simulink model "milestone3simulink"  (R2020a)
settings: Solver=VariableStepAuto  StartTime=0.0  StopTime=500  RelTol=1e-3
values from neighbouring files (symbols this model uses):
  ac = A-bc*C    [milestone3constants.m]
  alpha_initial = -theta+atan2(dy,dx)    [milestone3constants.m]
  bc = bc_1'    [milestone3constants.m]
  Beq = 0.2963    [milestone3constants.m]
  beta_initial = -theta-alpha_initial    [milestone3constants.m]
  del_weight = 1    [milestone3constants.m]
  g = 9.81    [milestone3constants.m]
  Jeq = 0.01802    [milestone3constants.m]
  k = place(A,B,p)    [milestone3constants.m]
  k_z = B-bc*D    [milestone3constants.m]
  Kb = 2.2179e-3    (= 0.0022179)    [milestone3constants.m]
  Keq = 0.74    [milestone3constants.m]
  mu = 0.01    [milestone3constants.m]
  p_initial = sqrt(dx^2+dy^2)    [milestone3constants.m]
  pick_up = 100    [milestone3constants.m]
  r = 0.037    [milestone3constants.m]
  ra = 7.4    [milestone3constants.m]
  un = [0 0]    [milestone3constants.m]
  v_i = 0    [milestone3constants.m]
  v_o = 0    [milestone3constants.m]
  wl_initial = 0    [milestone3constants.m]
  Wr = 0.18    [milestone3constants.m]
  wr_initial = 0    [milestone3constants.m]
  x_initial = [p_initial alpha_initial beta_initial 3.3275 3.3275]    [milestone3constants.m]
  yn = zeros(1,3)    [milestone3constants.m]
settings Model: Creator=oliviaball  LastModifiedBy=oliviaball
settings DataIOCC: MaxDataPoints=400  ReturnWorkspaceOutputs=off
settings DebuggingCC: ArithmeticOperatorsInVariantConditions=warning
settings SFSimCC: CustomCodeUndefinedFunction=UseInterfaceOnly

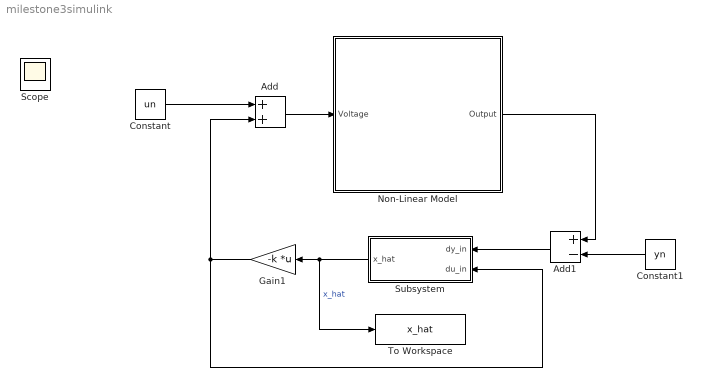
== system milestone3simulink ==
  Add : Sum
  Add1 : Sum  Inputs=+-
  Constant : Constant  Value=un
  Constant1 : Constant  Value=yn
  Gain1 : Gain  Gain=-k  Multiplication=Matrix(K*u)
  Non-Linear Model : Subsystem
  Subsystem : Subsystem
  To Workspace : ToWorkspace  VariableName=x_hat  SaveFormat=Timeseries  SampleTime=-1
  Scope : Scope
  wires:
  Add/1 -> Non-Linear Model/1(Voltage)
  Gain1/1 -> Subsystem/2(du_in), Add/2
  Constant/1 -> Add/1
  Non-Linear Model/1(Output) -> Add1/1
  Constant1/1 -> Add1/2
  Subsystem/1(x_hat) -> To Workspace/1, Gain1/1  "x_hat"
  Add1/1 -> Subsystem/1(dy_in)

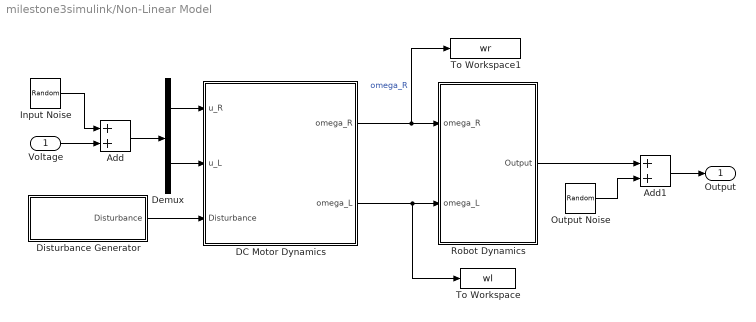
== system milestone3simulink/Non-Linear Model ==
  Voltage : Inport
  Add : Sum
  Add1 : Sum
  DC Motor Dynamics : Subsystem
  Demux : Demux  Outputs=2
  "Disturbance Generator " : Subsystem
  Input Noise : RandomNumber  Variance=v_i  SampleTime=1
  Output Noise : RandomNumber  Variance=v_o  SampleTime=50
  Robot Dynamics : Subsystem
  To Workspace : ToWorkspace  VariableName=wl  SaveFormat=Timeseries  SampleTime=-1
  To Workspace1 : ToWorkspace  VariableName=wr  SaveFormat=Timeseries  SampleTime=-1
  Output : Outport
  wires:
  "Disturbance Generator "/1("Disturbance ") -> DC Motor Dynamics/3(Disturbance)
  Demux/2 -> DC Motor Dynamics/2(u_L)
  Demux/1 -> DC Motor Dynamics/1(u_R)
  Add/1 -> Demux/1
  Voltage/1 -> Add/2
  Input Noise/1 -> Add/1
  DC Motor Dynamics/2(omega_L) -> Robot Dynamics/2(omega_L), To Workspace/1
  DC Motor Dynamics/1(omega_R) -> Robot Dynamics/1(omega_R), To Workspace1/1  "omega_R"
  Add1/1 -> Output/1
  Robot Dynamics/1(Output) -> Add1/1
  Output Noise/1 -> Add1/2

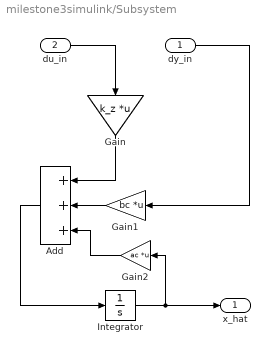
== system milestone3simulink/Subsystem ==
  dy_in : Inport
  du_in : Inport  Port=2
  Add : Sum  Inputs=+++
  Gain : Gain  Gain=k_z  Multiplication=Matrix(K*u)
  Gain1 : Gain  Gain=bc  Multiplication=Matrix(K*u)
  Gain2 : Gain  Gain=ac  Multiplication=Matrix(K*u)
  Integrator : Integrator  InitialCondition=x_initial
  x_hat : Outport
  wires:
  du_in/1 -> Gain/1
  Gain/1 -> Add/1
  Gain1/1 -> Add/2
  dy_in/1 -> Gain1/1
  Gain2/1 -> Add/3
  Add/1 -> Integrator/1
  Integrator/1 -> x_hat/1, Gain2/1

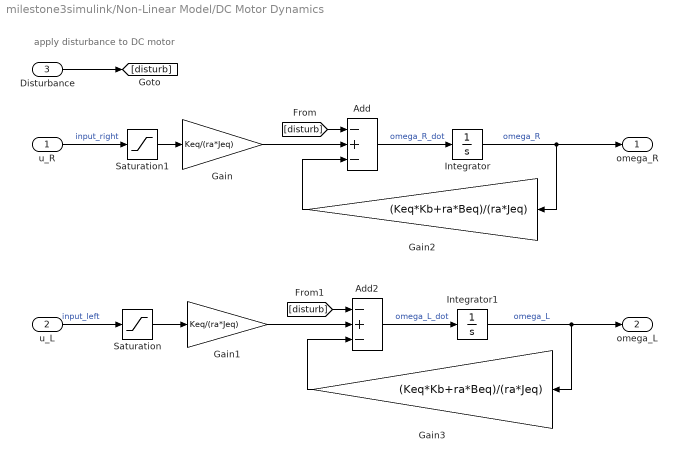
== system milestone3simulink/Non-Linear Model/DC Motor Dynamics ==
  note: apply disturbance to DC motor
  u_R : Inport
  u_L : Inport  Port=2
  Disturbance : Inport  Port=3
  Add : Sum  Inputs=-+-
  Add2 : Sum  Inputs=-+-
  Gain : Gain  Gain=Keq/(ra*Jeq)
  Gain1 : Gain  Gain=Keq/(ra*Jeq)
  Gain2 : Gain  Gain=(Keq*Kb+ra*Beq)/(ra*Jeq)
  Gain3 : Gain  Gain=(Keq*Kb+ra*Beq)/(ra*Jeq)
  Integrator : Integrator  InitialCondition=wr_initial
  Integrator1 : Integrator  InitialCondition=wl_initial
  Saturation : Saturate  UpperLimit=10  LowerLimit=-10
  Saturation1 : Saturate  UpperLimit=10  LowerLimit=-10
  omega_R : Outport  VectorParamsAs1DForOutWhenUnconnected=off
  omega_L : Outport  Port=2  VectorParamsAs1DForOutWhenUnconnected=off
  wires:
  u_R/1 -> Saturation1/1  "input_right"
  Add/1 -> Integrator/1  "omega_R_dot"
  Integrator/1 -> omega_R/1, Gain2/1  "omega_R"
  Add2/1 -> Integrator1/1  "omega_L_dot"
  Integrator1/1 -> omega_L/1, Gain3/1  "omega_L"
  u_L/1 -> Saturation/1  "input_left"
  Gain3/1 -> Add2/3
  Gain1/1 -> Add2/2
  Gain2/1 -> Add/3
  Gain/1 -> Add/2
  [disturb] -> Add/1
  Disturbance/1 -> [disturb]
  [disturb] -> Add2/1
  Saturation/1 -> Gain1/1
  Saturation1/1 -> Gain/1

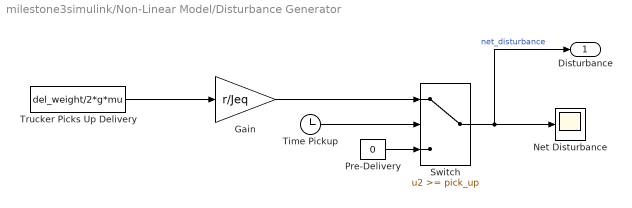
== system milestone3simulink/Non-Linear Model/Disturbance Generator  ==
  Gain : Gain  Gain=r/Jeq
  "Net Disturbance " : Scope
  Pre-Delivery : Constant  Value=0
  Switch : Switch  Threshold=pick_up
  Time Pickup : Clock
  Trucker Picks Up Delivery : Constant  Value=del_weight/2*g*mu
  "Disturbance " : Outport  VectorParamsAs1DForOutWhenUnconnected=off
  wires:
  Time Pickup/1 -> Switch/2
  Pre-Delivery/1 -> Switch/3
  Switch/1 -> "Disturbance "/1, "Net Disturbance "/1  "net_disturbance"
  Gain/1 -> Switch/1
  Trucker Picks Up Delivery/1 -> Gain/1

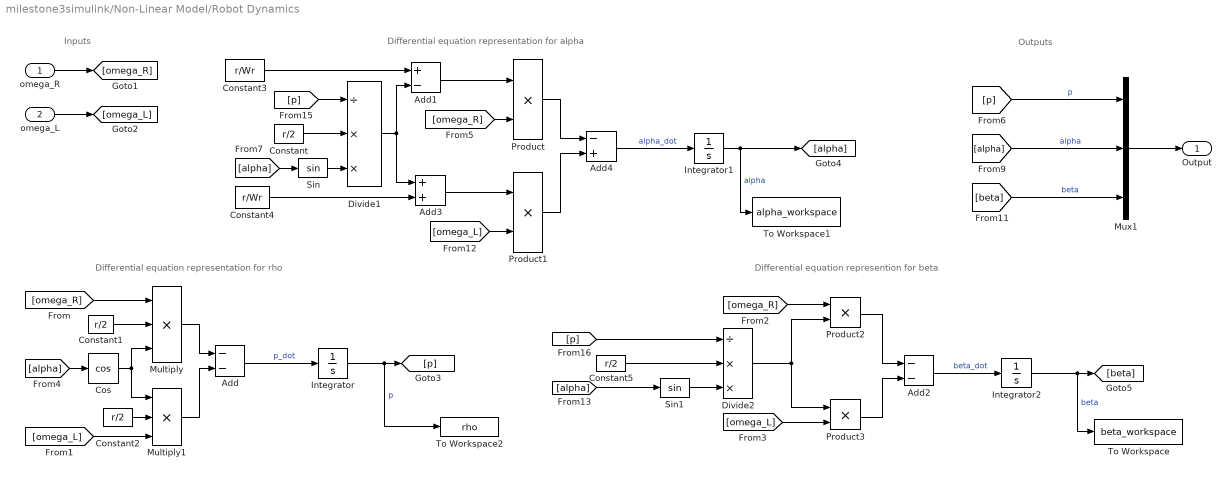
== system milestone3simulink/Non-Linear Model/Robot Dynamics ==
  note: Inputs
  note: Outputs
  note: Differential equation representation for rho
  note: Differential equation represention for beta
  note: Differential equation representation for alpha
  omega_R : Inport
  omega_L : Inport  Port=2
  Add : Sum  Inputs=--
  Add1 : Sum  Inputs=+-
  Add2 : Sum  Inputs=--
  Add3 : Sum
  Add4 : Sum  Inputs=-+
  Constant{,1..2,5} (4 alike) : Constant  Value=r/2
  Constant3 : Constant  Value=r/Wr
  Constant4 : Constant  Value=r/Wr
  Cos : Trigonometry  Operator=cos
  Divide1 : Product  Inputs=/**
  Divide2 : Product  Inputs=/**
  Integrator : Integrator  InitialCondition=p_initial
  Integrator1 : Integrator  InitialCondition=alpha_initial
  Integrator2 : Integrator  InitialCondition=beta_initial
  Multiply : Product  Inputs=3
  Multiply1 : Product  Inputs=3
  Mux1 : Mux  Inputs=3
  Product{,1..3} (4 alike) : Product
  Sin : Trigonometry
  Sin1 : Trigonometry
  To Workspace : ToWorkspace  VariableName=beta_workspace  SaveFormat=Timeseries  SampleTime=-1
  To Workspace1 : ToWorkspace  VariableName=alpha_workspace  SaveFormat=Timeseries  SampleTime=-1
  To Workspace2 : ToWorkspace  VariableName=rho  SaveFormat=Timeseries  SampleTime=-1
  Output : Outport
  wires:
  omega_R/1 -> [omega_R]
  omega_L/1 -> [omega_L]
  Sin/1 -> Divide1/3
  Integrator/1 -> To Workspace2/1, [p]  "p"
  Integrator1/1 -> [alpha], To Workspace1/1  "alpha"
  Add2/1 -> Integrator2/1  "beta_dot"
  Add4/1 -> Integrator1/1  "alpha_dot"
  Multiply1/1 -> Add/2
  Multiply/1 -> Add/1
  [alpha] -> Cos/1
  Constant2/1 -> Multiply1/2
  [alpha] -> Sin/1
  Add/1 -> Integrator/1  "p_dot"
  Integrator2/1 -> To Workspace/1, [beta]  "beta"
  Cos/1 -> Multiply/3, Multiply1/1
  [omega_L] -> Product1/2
  [alpha] -> Sin1/1
  Sin1/1 -> Divide2/3
  [p] -> Divide1/1
  Divide1/1 -> Add3/1, Add1/2
  [p] -> Divide2/1
  [omega_R] -> Multiply/1
  Constant1/1 -> Multiply/2
  [omega_L] -> Multiply1/3
  Constant/1 -> Divide1/2
  Constant3/1 -> Add1/1
  Add1/1 -> Product/1
  [omega_R] -> Product/2
  Constant4/1 -> Add3/2
  Add3/1 -> Product1/1
  Product/1 -> Add4/1
  Product1/1 -> Add4/2
  Constant5/1 -> Divide2/2
  [omega_R] -> Product2/1
  Divide2/1 -> Product2/2, Product3/1
  [omega_L] -> Product3/2
  Product2/1 -> Add2/1
  Product3/1 -> Add2/2
  [p] -> Mux1/1  "p"
  [alpha] -> Mux1/2  "alpha"
  [beta] -> Mux1/3  "beta"
  Mux1/1 -> Output/1
